simulink model "handmade_motor_inertial_load"  (R2024b)
settings: Solver=ode45  StartTime=0.0  StopTime=10.0  RelTol=1e-3
values from neighbouring files (symbols this model uses):
  Beq = 2.0e-6    (= 2e-06)    [Parameters_estimation.m]    (also in Real_time_parameter_estimation.m = (data.Beq_hat_pos + data.Beq_hat_neg)/2; data.m; real-time-estimation.mat = 1.22371676185e-06)
  Jeq_hat = avg/N_periods    (= 0)    [Parameters_estimation.m]    (also in Real_time_parameter_estimation.m; real-time-estimation.mat = 5.73206536577e-05)
  rads2rpm = 60/2/pi    (= 9.54929658551)    [Init.m]    (also in ModelParams.m; data.m; load_params_inertial_case.m)
  tau_sf = 1.0e-2    (= 0.01)    [Parameters_estimation.m]    (also in Real_time_parameter_estimation.m = (abs(data.tau_sf_pos)+abs(data.tau_sf_neg))/2; data.m; real-time-estimation.mat = 0.00570915114298)
undefined symbols (not defined in the file or in its folder): daq, drv, k_drv, Ke, Kt, mot, N, Req, sens, T_drv
settings Model: Creator=lucag  LastModifiedBy=lucag

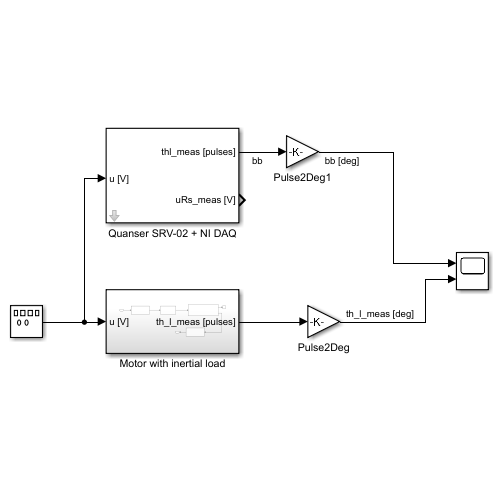
[thumbnail: Simulink's stored preview of the top-level diagram]
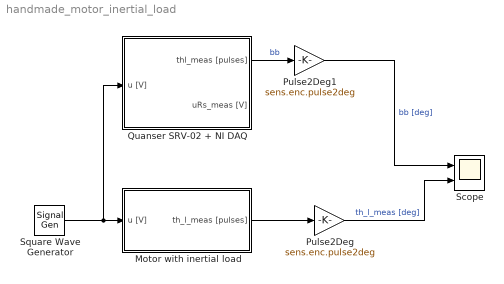
== system handmade_motor_inertial_load ==
  Motor with inertial load : Subsystem
  Pulse2Deg : Gain  Gain=sens.enc.pulse2deg
  Pulse2Deg1 : Gain  Gain=sens.enc.pulse2deg
  Quanser SRV-02 + NI DAQ : Subsystem  mask(Quanser SRV-02 (with inertial load) + NI DAQ){Ts=0.001, fricType=Coulomb + viscous}
      mask prompts: Ts "NI DAQ Sample Time:"; fricType "Friction model"
      mask help: Quanser SRV-02 (with inertial load) + NI DAQ model.
      mask init:
      | %%  Sensors data
      | 
      | %   shunt resistor
      | sens.curr.Rs = 0.5;                         %   resistance [Ohm]   
      | sens.curr.uRs_std = 0.01;                   %   voltage noise standard dev [V]                           
      | sens.curr.uRs_var = sens.curr.uRs_std^2;	%   voltage noise variance [V^2]
      | 
      | %   Hewlett-Packard HEDS-5540#A06 optical encoder
      | sens.enc.ppr = 500*4;                       %   pulses per rotation
      | sens.enc.pulse2deg = 360/sens.enc.ppr;      %   [pulses] -> [deg]
      | sens.enc.pulse2rad = 2*pi/sens.enc.ppr;     %   [pulses] -> [rad]
      | sens.enc.deg2pulse = sens.enc.ppr/360;      %   [deg] -> [pulses]
      | sens.enc.rad2pulse = sens.enc.ppr/2/pi;     %   [rad] -> [pulses]
      | 
      | 
      | %%  Data acquisition board (daq) data
      | 
      | %   NI PCI-6221 DAC data
      | daq.dac.bits = 16;                                  %   resolution (bits)
      | daq.dac.fs   = 10;                                  %   full scale 
      | daq.dac.q    = 2*daq.dac.fs/(2^daq.dac.bits-1);     %	quantization
      | 
      | %   NI PCI-6221 ADC data
      | daq.adc.bits = 16;                                  %   resolution (bits)
      | daq.adc.fs   = 10;                                  %   full scale (as set in SLDRT Analog Input block)
      | daq.adc.q    = 2*daq.adc.fs/(2^daq.adc.bits-1);     %   quantization
      mask Help:
      | Riccardo Antonello (antonello@dei.unipd.it)
      | 
      | April 24, 2020
      | 
      | Dept. of Information Engineering, University of Padova
      mask TypeOptions fricType: Coulomb + viscous | Karnopp
  Scope : Scope  NumInputPorts=2
  Square Wave Generator : SignalGenerator  WaveForm=square  Amplitude=10  Units=rad/sec
  wires:
  Square Wave Generator/1 -> Quanser SRV-02 + NI DAQ/1(u [V]), Motor with inertial load/1(u [V])
  Pulse2Deg/1 -> Scope/2  "th_l_meas [deg]"
  Motor with inertial load/1(th_l_meas [pulses]) -> Pulse2Deg/1
  Quanser SRV-02 + NI DAQ/1(thl_meas [pulses]) -> Pulse2Deg1/1  "bb"
  Pulse2Deg1/1 -> Scope/1  "bb [deg]"

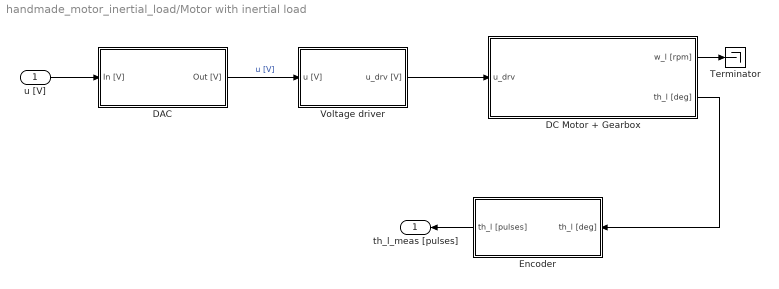
== system handmade_motor_inertial_load/Motor with inertial load ==
  u [V] : Inport
  DAC : Subsystem
  DC Motor + Gearbox : Subsystem
  Encoder : Subsystem
  Terminator : Terminator
  Voltage driver : Subsystem
  th_l_meas [pulses] : Outport
  wires:
  DC Motor + Gearbox/2(th_l [deg]) -> Encoder/1(th_l [deg])
  DC Motor + Gearbox/1(w_l [rpm]) -> Terminator/1
  Encoder/1(th_l [pulses]) -> th_l_meas [pulses]/1
  u [V]/1 -> DAC/1(In [V])
  Voltage driver/1(u_drv [V]) -> DC Motor + Gearbox/1(u_drv)
  DAC/1(Out [V]) -> Voltage driver/1(u [V])  "u [V]"

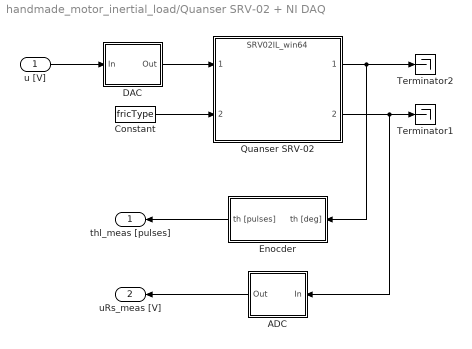
== system handmade_motor_inertial_load/Quanser SRV-02 + NI DAQ ==
  u [V] : Inport
  ADC : Subsystem
  Constant : Constant  Value=fricType
  DAC : Subsystem
  Enocder : Subsystem
  Quanser SRV-02 : ModelReference  ModelNameDialog=SRV02IL_win64.slxp  ModelReferenceVersion=1.44  CopyOfModelProtected=on
  Terminator1 : Terminator
  Terminator2 : Terminator
  thl_meas [pulses] : Outport
  uRs_meas [V] : Outport  Port=2
  wires:
  Enocder/1(th [pulses]) -> thl_meas [pulses]/1
  ADC/1(Out) -> uRs_meas [V]/1
  DAC/1(Out) -> Quanser SRV-02/1
  Quanser SRV-02/2 -> ADC/1(In), Terminator1/1
  u [V]/1 -> DAC/1(In)
  Quanser SRV-02/1 -> Enocder/1(th [deg]), Terminator2/1
  Constant/1 -> Quanser SRV-02/2

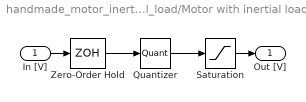
== system handmade_motor_inertial_load/Motor with inertial load/DAC ==
  In [V] : Inport
  Quantizer : Quantizer  QuantizationInterval=daq.dac.q
  Saturation : Saturate  UpperLimit=daq.dac.fs  LowerLimit=-daq.dac.fs
  Zero-Order Hold : ZeroOrderHold  SampleTime=1e-3
  Out [V] : Outport
  wires:
  Saturation/1 -> Out [V]/1
  Zero-Order Hold/1 -> Quantizer/1
  Quantizer/1 -> Saturation/1
  In [V]/1 -> Zero-Order Hold/1

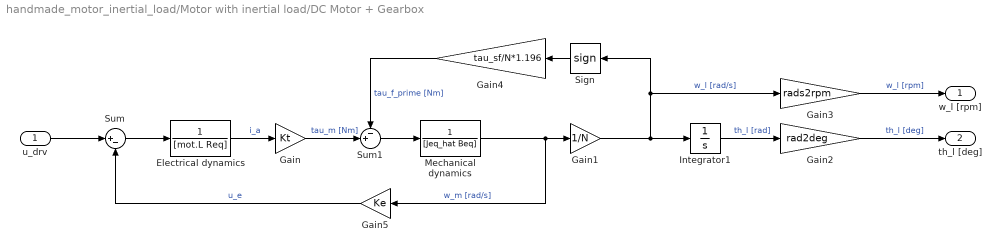
== system handmade_motor_inertial_load/Motor with inertial load/DC Motor + Gearbox ==
  u_drv : Inport
  Electrical dynamics : TransferFcn  Denominator=[mot.L Req]
  Gain : Gain  Gain=Kt
  Gain1 : Gain  Gain=1/N
  Gain2 : Gain  Gain=rad2deg
  Gain3 : Gain  Gain=rads2rpm
  Gain4 : Gain  Gain=tau_sf/N*1.196
  Gain5 : Gain  Gain=Ke
  Integrator1 : Integrator
  Mechanical dynamics : TransferFcn  Denominator=[Jeq_hat Beq]
  Sign : Signum  ZeroCross=off
  Sum : Sum  Inputs=|+-
  Sum1 : Sum  Inputs=-+|
  w_l [rpm] : Outport
  th_l [deg] : Outport  Port=2
  wires:
  Integrator1/1 -> Gain2/1  "th_l [rad]"
  Gain5/1 -> Sum/2  "u_e"
  Gain1/1 -> Sign/1, Gain3/1, Integrator1/1  "w_l [rad/s]"
  Electrical dynamics/1 -> Gain/1  "i_a"
  Sign/1 -> Gain4/1
  Sum/1 -> Electrical dynamics/1
  Sum1/1 -> Mechanical dynamics/1
  Gain/1 -> Sum1/2  "tau_m [Nm]"
  Gain3/1 -> w_l [rpm]/1  "w_l [rpm]"
  Mechanical dynamics/1 -> Gain5/1, Gain1/1  "w_m [rad/s]"
  Gain2/1 -> th_l [deg]/1  "th_l [deg]"
  u_drv/1 -> Sum/1
  Gain4/1 -> Sum1/1  "tau_f_prime [Nm]"

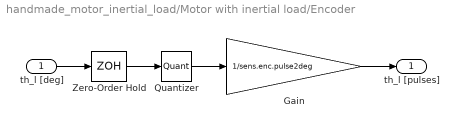
== system handmade_motor_inertial_load/Motor with inertial load/Encoder ==
  th_l [deg] : Inport
  Gain : Gain  Gain=1/sens.enc.pulse2deg
  Quantizer : Quantizer  QuantizationInterval=sens.enc.pulse2deg
  Zero-Order Hold : ZeroOrderHold  SampleTime=1e-3
  th_l [pulses] : Outport
  wires:
  th_l [deg]/1 -> Zero-Order Hold/1
  Quantizer/1 -> Gain/1
  Zero-Order Hold/1 -> Quantizer/1
  Gain/1 -> th_l [pulses]/1

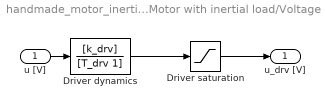
== system handmade_motor_inertial_load/Motor with inertial load/Voltage driver ==
  u [V] : Inport
  Driver dynamics : TransferFcn  Numerator=[k_drv]  Denominator=[T_drv 1]
  Driver saturation : Saturate  UpperLimit=drv.outmax  LowerLimit=-drv.outmax
  u_drv [V] : Outport
  wires:
  Driver dynamics/1 -> Driver saturation/1
  Driver saturation/1 -> u_drv [V]/1
  u [V]/1 -> Driver dynamics/1

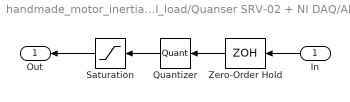
== system handmade_motor_inertial_load/Quanser SRV-02 + NI DAQ/ADC ==
  In : Inport
  Quantizer : Quantizer  QuantizationInterval=daq.adc.q
  Saturation : Saturate  UpperLimit=daq.adc.fs  LowerLimit=-daq.adc.fs
  Zero-Order Hold : ZeroOrderHold  SampleTime=Ts
  Out : Outport
  wires:
  Saturation/1 -> Out/1
  In/1 -> Zero-Order Hold/1
  Quantizer/1 -> Saturation/1
  Zero-Order Hold/1 -> Quantizer/1

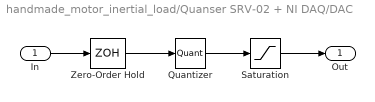
== system handmade_motor_inertial_load/Quanser SRV-02 + NI DAQ/DAC ==
  In : Inport
  Quantizer : Quantizer  QuantizationInterval=daq.dac.q
  Saturation : Saturate  UpperLimit=daq.dac.fs  LowerLimit=-daq.dac.fs
  Zero-Order Hold : ZeroOrderHold  SampleTime=Ts
  Out : Outport
  wires:
  Quantizer/1 -> Saturation/1
  In/1 -> Zero-Order Hold/1
  Zero-Order Hold/1 -> Quantizer/1
  Saturation/1 -> Out/1

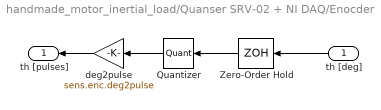
== system handmade_motor_inertial_load/Quanser SRV-02 + NI DAQ/Enocder ==
  th [deg] : Inport
  Quantizer : Quantizer  QuantizationInterval=sens.enc.pulse2deg
  Zero-Order Hold : ZeroOrderHold  SampleTime=Ts
  deg2pulse : Gain  Gain=sens.enc.deg2pulse
  th [pulses] : Outport
  wires:
  Quantizer/1 -> deg2pulse/1
  th [deg]/1 -> Zero-Order Hold/1
  Zero-Order Hold/1 -> Quantizer/1
  deg2pulse/1 -> th [pulses]/1
